simulink model "callFunctionSubsystem"  (R2018a)
settings: Solver=FixedStepDiscrete  StartTime=0.0  StopTime=inf  FixedStep=0.2  RelTol=1e-3
settings Model: Creator=Ayman_Elgammal  LastModifiedBy=Ayman_Elgammal

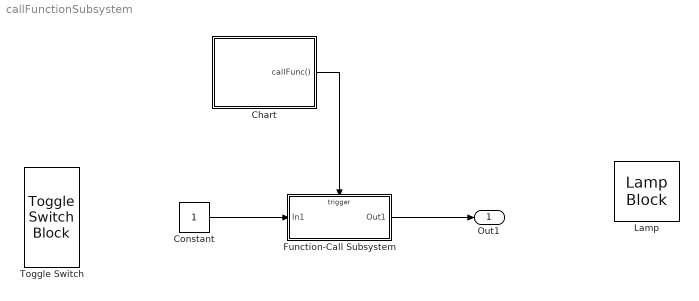
== system callFunctionSubsystem ==
  Chart : Stateflow chart  TreatAsAtomicUnit=on
  Constant : Constant
  Function-Call Subsystem : Subsystem  TreatAsAtomicUnit=on
  Lamp : LampBlock  WebBlockId=7
  Toggle Switch : ToggleSwitchBlock  WebBlockId=8
      settings: Values={{'Off', 'On'}, [0 1]}
  Out1 : Outport
  wires:
  Constant/1 -> Function-Call Subsystem/1(In1)
  Chart/1(callFunc()) -> Function-Call Subsystem/Trigger
  Function-Call Subsystem/1(Out1) -> Out1/1

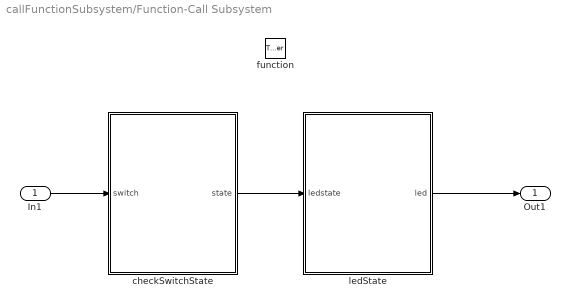
== system callFunctionSubsystem/Function-Call Subsystem ==
  In1 : Inport
  function : TriggerPort  TriggerType=function-call  VariantControl=Variant
  checkSwitchState : Stateflow chart  TreatAsAtomicUnit=on
  ledState : Stateflow chart  TreatAsAtomicUnit=on
  Out1 : Outport
  wires:
  In1/1 -> checkSwitchState/1(switch)
  checkSwitchState/1(state) -> ledState/1(ledstate)
  ledState/1(led) -> Out1/1

== stateflow chart callFunctionSubsystem/Function-Call Subsystem/checkSwitchState ==
  (default) -> (junction 7) : % check_switch
  (junction 7) -> (junction 8) [order 1] : [switch == 1]
  (junction 7) -> (junction 9) [order 2] : {state =  0;}
  (junction 8) -> (junction 10) : {state = 1;}
  (junction 10) -> (junction 9)
  (junction 9) -> (junction 11)
  data: switch input double; state output double

== stateflow chart callFunctionSubsystem/Function-Call Subsystem/ledState ==
  (default) -> (junction 7) : % ledState
  (junction 7) -> (junction 8) [order 1] : [ledstate == 1]
  (junction 7) -> (junction 9) [order 2] : {led = 0;}
  (junction 8) -> (junction 10) : {led = 1;}
  (junction 10) -> (junction 9)
  (junction 9) -> (junction 11)
  data: ledstate input; led output

== stateflow chart callFunctionSubsystem/Chart ==
  state callFunction
    en:
    du:
    ex:
  (default) -> callFunction
  callFunction -> callFunction : [after(5,msec)]{callFunc;}
  events: callFunc output FUNCTION_CALL_EVENT
